simulink model "PedBridge_sim"  (R2022a)
settings: Solver=ode4  StartTime=t_init  StopTime=t_final  FixedStep=t_step  RelTol=1e-3
values from neighbouring files (symbols this model uses):
  As = [zeros(n_modos) eye(n_modos); -Me\Ke -Me\Ce]    [SpaceState_bridge.m]
  Bs = [zeros(n_modos); Me\Ge]    [SpaceState_bridge.m]
  Cs = [eye(n_modos) zeros(n_modos) ; zeros(n_modos) eye(n_modos); -Me\Ke -Me\Ce]    [SpaceState_bridge.m]
  Ds = [zeros(n_modos) ; zeros(n_modos); Me\Ge]    [SpaceState_bridge.m]
  posi = [(0:1:20).' ; (19:-1:0).']    [FunctionTesting.m]
  psi_posi = zeros(t_length,n_modos,pd_length)    [NewPedestrianProperties.m]    (also in NewPedestrianPropertiesGenerator.m)
undefined symbols (not defined in the file or in its folder): ai, lambdai, mi, wi
settings Model: Creator=LEGION  LastModifiedBy=LEGION

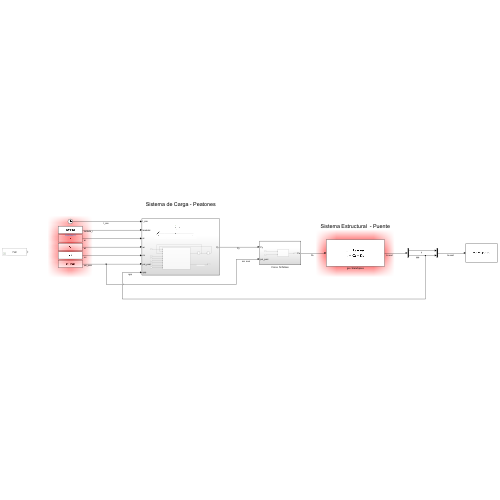
[thumbnail: Simulink's stored preview of the top-level diagram]
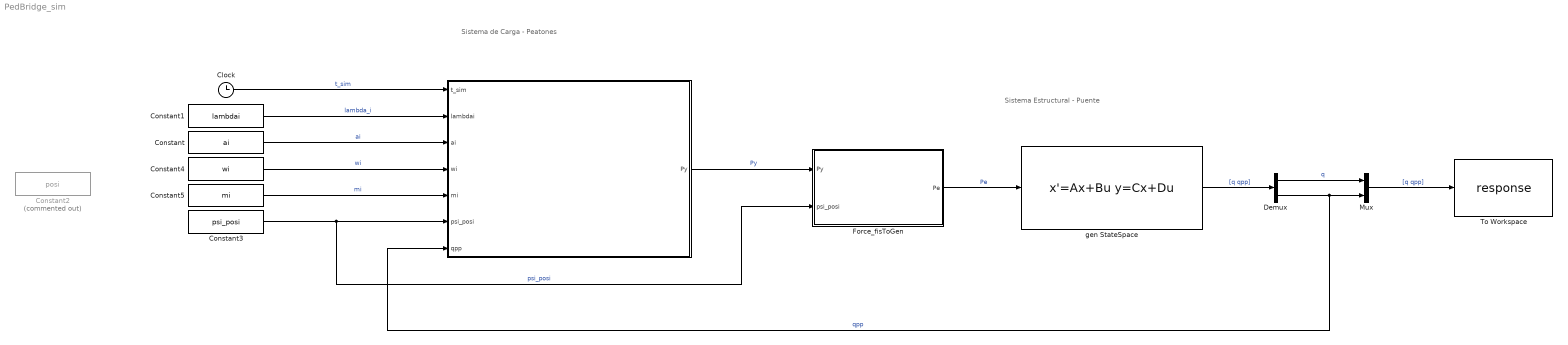
== system PedBridge_sim ==
  note: Sistema de Carga - Peatones
  note: Sistema Estructural - Puente
  " " : Subsystem
  Clock : Clock
  Constant : Constant  Value=ai  SampleTime=-1
  Constant1 : Constant  Value=lambdai  SampleTime=-1
  Constant2 : Constant  Commented=on  Value=posi  SampleTime=-1
  Constant3 : Constant  Value=psi_posi  SampleTime=-1
  Constant4 : Constant  Value=wi  SampleTime=-1
  Constant5 : Constant  Value=mi  SampleTime=-1
  Demux : Demux  Outputs=2
  Force_fisToGen : Subsystem
  Mux : Mux  Inputs=2
  To Workspace : ToWorkspace  VariableName=response  SaveFormat=Timeseries  SampleTime=-1
  gen StateSpace : StateSpace  A=As  B=Bs  C=Cs  D=Ds  InitialCondition=0
  wires:
  " "/1(Py) -> Force_fisToGen/1(Py)  "Py"
  Force_fisToGen/1(Pe) -> gen StateSpace/1  "Pe"
  Constant3/1 -> Force_fisToGen/2(psi_posi), " "/6(psi_posi)  "psi_posi"
  Constant5/1 -> " "/5(mi)  "mi"
  Constant4/1 -> " "/4(wi)  "wi"
  Constant/1 -> " "/3(ai)  "ai"
  Constant1/1 -> " "/2(lambdai)  "lambda_i"
  Clock/1 -> " "/1(t_sim)  "t_sim"
  gen StateSpace/1 -> Demux/1  "[q qpp]"
  Demux/1 -> Mux/1  "q"
  Demux/2 -> Mux/2, " "/7(qpp)  "qpp"
  Mux/1 -> To Workspace/1  "[q qpp]"

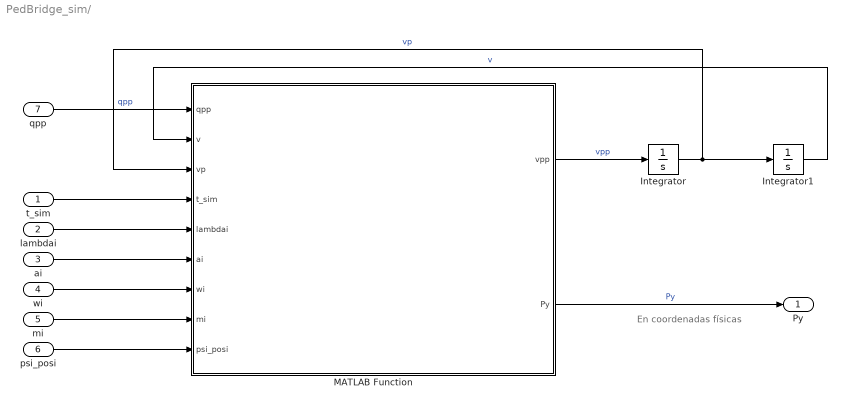
== system PedBridge_sim/  ==
  note: En coordenadas físicas
  t_sim : Inport
  lambdai : Inport  Port=2
  ai : Inport  Port=3
  wi : Inport  Port=4
  mi : Inport  Port=5
  psi_posi : Inport  Port=6
  qpp : Inport  Port=7
  Integrator : Integrator
  Integrator1 : Integrator
  MATLAB Function : MATLAB Function  TreatAsAtomicUnit=on
  Py : Outport
  wires:
  qpp/1 -> MATLAB Function/1(qpp)  "qpp"
  MATLAB Function/2(Py) -> Py/1  "Py"
  MATLAB Function/1(vpp) -> Integrator/1  "vpp"
  Integrator/1 -> MATLAB Function/3(vp), Integrator1/1  "vp"
  Integrator1/1 -> MATLAB Function/2(v)  "v"
  lambdai/1 -> MATLAB Function/5(lambdai)
  ai/1 -> MATLAB Function/6(ai)
  wi/1 -> MATLAB Function/7(wi)
  mi/1 -> MATLAB Function/8(mi)
  psi_posi/1 -> MATLAB Function/9(psi_posi)
  t_sim/1 -> MATLAB Function/4(t_sim)

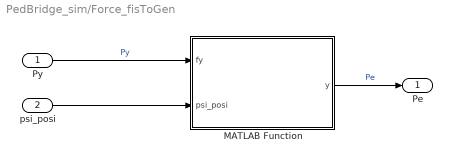
== system PedBridge_sim/Force_fisToGen ==
  Py : Inport
  psi_posi : Inport  Port=2
  MATLAB Function : MATLAB Function  TreatAsAtomicUnit=on
  Pe : Outport
  wires:
  Py/1 -> MATLAB Function/1(fy)  "Py"
  psi_posi/1 -> MATLAB Function/2(psi_posi)
  MATLAB Function/1(y) -> Pe/1  "Pe"

== matlab function PedBridge_sim/Force_fisToGen/MATLAB Function ==
  data: fy input; y output; psi_posi input
function y = fcn(fy, psi_posi)
% Determinar Pe, entrada para sistema estructural (puente) en
% representación espacio estado de la viga equivalente cuya dinámica en 
% todo el largo se obtiene por el método de modos asumidos

% Pe = sum_n(sum_i(Py_i.*psi_n_pos_i))

== matlab function PedBridge_sim/ /MATLAB Function ==
  data: qpp input; v input; vp input; t_sim input; lambdai input; ai input; wi input; mi input; vpp output; Py output; psi_posi input
function [vpp, Py] = fcn(qpp, v, vp, t_sim, lambdai, ai, wi, mi,psi_posi)
%% Generar Py, fuerza de todos los peatones

% INPUTS
% qpp:  Vector fila de la aceleración en coordenadas físicas que experimenta cada peatón
% v:    Desplazamiento

% OUTSPUTS


% COMENTARIOS
% en una MATLAB FUNCTION yo no recorro en tiempo, se asume que solo se ve
% una franja de tiempo
%% Previous Data
pd_length = length(mi);
n_modos = size(qpp,2);

%% Generar ypp
% Hay que generar la aceleración que tiene el peatón en el tiempo "t"
% para ello se compone la 
ypp_ = zeros(pd_length,n_modos);
ypp = zeros(pd_length,1);
for i = 1:pd_length                                                        % Para cada peatón
    for n = 1:n_modos
        ypp_(i,n) = psi_posi(i,n)*qpp(n);
    end
    ypp(i,1) = sum(ypp_(i,:),2);
end

%% Resolver dinámica del peatón
% Modelo de Belykh et al 2017
vpp = zeros(pd_length,1);
for i = 1:pd_length
    fvdv = lambdai(i)*(vp(i)^2 + v(i)^2 - ai(i)^2)*vp(i) + wi(i)^2*v(i);    % (Eq.5)
    vpp(i) = -yppi(i) - fvdv;                                               % (Eq.1) 
end

%% Generar Py
% La fuerza que genera cada peatón (no se adjunta la posición del peatón)
Py = mi*vpp;


%% no van con end
